simulink model "rlKinovaBallBalance"  (R2024a)
settings: Solver=ode15s  StartTime=0.0  StopTime=200  RelTol=1e-3  AbsTol=1e-3
undefined symbols (not defined in the file): ball, Control, L1, L2, L3, LS1, LS3, max_torque, plate, R1, R1_q0, R2, R2_q0, R3, R3_q0, R4_q0, R5_q0, Rover, rover_path, RS1, RS3, U0, X, Y, Z
libraries: sm_lib x227, nesl_utility x104, fl_lib x85, sdl_lib x20, nesl_utility_internal x17, ee_lib x10, mars_rover_lib x7, simulink x3, slpidlib x2, batteryecm_lib x2, robotalgslib x1, rllib x1
(part 3 of 10)

== system rlKinovaBallBalance/Kinova Ball Balance/7 DOF Manipulator/base_link ==
  Actuator1_AxisTransform : sm_lib/Frames and Transforms/Rigid Transform  RotationMethod=ArbitraryAxis  FollAlignAxisA=+X  BaseAlignAxisA=+Y  FollAlignAxisB=+Y  BaseAlignAxisB=+Z  RotationStandardAxis=+Z  RotationAngle=0  RotationAngleUnits=rad  RotationArbitraryAxis=[1, 0, 0]  RotationSequenceAxes=FollowerAxes  RotationSequence=XYX  RotationSequenceAngles=[0 0 0]  RotationSequenceAnglesUnits=deg  RotationMatrix=[1 0 0; 0 1 0; 0 0 1]  Quaternion=[1 0 0 0]  TranslationMethod=Cartesian  TranslationCartesianOffset=[0, 0, 0]  TranslationCartesianOffsetUnits=m  TranslationStandardAxis=+Z  TranslationStandardOffset=0  TranslationStandardOffsetUnits=m  TranslationROffset=0  TranslationROffsetUnits=m  TranslationThetaOffset=0  TranslationThetaOffsetUnits=deg  TranslationZOffset=0  TranslationZOffsetUnits=m
  Actuator1_OriginTransform : sm_lib/Frames and Transforms/Rigid Transform  RotationMethod=RotationSequence  FollAlignAxisA=+X  BaseAlignAxisA=+Y  FollAlignAxisB=+Y  BaseAlignAxisB=+Z  RotationStandardAxis=+Z  RotationAngle=0.0  RotationAngleUnits=deg  RotationArbitraryAxis=[0 0 1]  RotationSequenceAxes=BaseAxes  RotationSequence=XYZ  RotationSequenceAngles=[-3.141585307179587, 0, 0]  RotationSequenceAnglesUnits=rad  RotationMatrix=[1 0 0; 0 1 0; 0 0 1]  Quaternion=[1 0 0 0]  TranslationMethod=Cartesian  TranslationCartesianOffset=[0, 0, 0.15643]  TranslationCartesianOffsetUnits=m  TranslationStandardAxis=+Z  TranslationStandardOffset=0  TranslationStandardOffsetUnits=m  TranslationROffset=0  TranslationROffsetUnits=m  TranslationThetaOffset=0  TranslationThetaOffsetUnits=deg  TranslationZOffset=0  TranslationZOffsetUnits=m
  Base Link : Subsystem  Variant=on  VariantControlMode=label  VariantControl=Choice  LabelModeActiveChoice=Choice_1
  ReferenceFrame : sm_lib/Frames and Transforms/Reference Frame
  F : PMIOPort  Side=Left
  F1 : PMIOPort  Port=2  Side=Right
  connections:
  Actuator1_AxisTransform/RConn1 -- F1/RConn1
  Actuator1_AxisTransform/LConn1 -- Actuator1_OriginTransform/RConn1
  F/RConn1 -- Actuator1_OriginTransform/LConn1 -- ReferenceFrame/RConn1 -- Base Link/RConn1

== system rlKinovaBallBalance/Kinova Ball Balance/7 DOF Manipulator/mount ==
  Cylindrical Solid : sm_lib/Body Elements/Cylindrical Solid  CylinderRadius=0.1  CylinderRadiusUnits=m  CylinderLength=0.01  CylinderLengthUnits=m  ExportEntireGeometry=off  InertiaType=CalculateFromGeometry  BasedOnType=Density  Density=1000  DensityUnits=kg/m^3  Mass=1  MassUnits=kg  CenterOfMass=[0 0 0]  CenterOfMassUnits=m  MomentsOfInertia=[1 1 1]  MomentsOfInertiaUnits=kg*m^2  ProductsOfInertia=[0 0 0]  ProductsOfInertiaUnits=kg*m^2  GraphicType=FromGeometry  MarkerShape=Sphere  MarkerSize=10  GraphicVisPropType=SimpleVisualProperties  GraphicDiffuseColor=[0.6 0.6 0.6]  GraphicOpacity=1.0  GraphicSpecularColor=[0.5 0.5 0.5 1.0]  GraphicAmbientColor=[0.15 0.15 0.15 1.0]  GraphicEmissiveColor=[0.0 0.0 0.0 1.0]  GraphicShininess=75  DoExposeReferenceFrame=off  SerializedFrames=<Frames><Frame><Id>Frame1</Id><Value><Name>F1</Name><Origin><Source>GeometricFeature</Source><FeatureName>top surface</FeatureName></Origin><PrimaryAxis><DefinedDirection>+Z</DefinedDirection><Source>ReferenceFrame</Source><SourceDirection>+Z</SourceDirection><FeatureName></FeatureName></PrimaryAxis><SecondaryAxis><DefinedDirection>+X</DefinedDirection><Source>ReferenceFrame</Source><SourceDirection>+X</SourceDirection><FeatureName></FeatureName></SecondaryAxis></Value></Frame><Frame><Id>Frame2</Id><Value><Name>F2</Name><Origin><Source>GeometricFeature</Source><FeatureName>bottom surface</FeatureName></Origin><PrimaryAxis><DefinedDirection>+Z</DefinedDirection><Source>ReferenceFrame</Source><SourceDirection>+Z</SourceDirection><FeatureName></FeatureName></PrimaryAxis><SecondaryAxis><DefinedDirection>+X</DefinedDirection><Source>ReferenceFrame</Source><SourceDirection>+X</SourceDirection><FeatureName></FeatureName></SecondaryAxis></Value></Frame></Frames>
  F : PMIOPort  Side=Right
  F1 : PMIOPort  Port=2  Side=Left
  connections:
  Cylindrical Solid/LConn1 -- F1/RConn1
  F/RConn1 -- Cylindrical Solid/RConn1

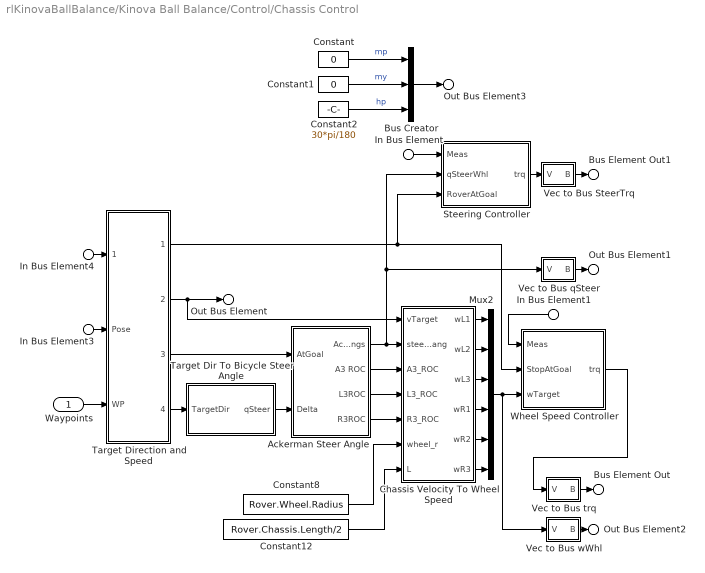
== system rlKinovaBallBalance/Kinova Ball Balance/Control/Chassis Control ==
  Waypoints : Inport
  In Bus Element1 : Inport  Port=2  PortName=Chassis  Element=Wheels.Drive
  In Bus Element : Inport  Port=2  PortName=Chassis  Element=Wheels.Steer
  In Bus Element3 : Inport  Port=3  PortName=Body  Element=Pose
  In Bus Element4 : Inport  Port=3  PortName=Body  Element=v
  Ackerman Steer Angle : Subsystem
  Bus Creator : BusCreator  Inputs=3
  Chassis Velocity To Wheel Speed : MATLAB Function  TreatAsAtomicUnit=on
  Constant : Constant  Value=0
  Constant1 : Constant  Value=0
  Constant12 : Constant  Value=Rover.Chassis.Length/2
  Constant2 : Constant  Value=30*pi/180
  Constant8 : Constant  Value=Rover.Wheel.Radius
  Mux2 : Mux  Inputs=6
  Steering Controller : Subsystem  mask{Kp=Control.Steer.Kp, Ki=Control.Steer.Ki, Kd=Control.Steer.Kd, N=Control.Steer.N, Ts_Targetq=Control.Steer.FiltTargetq, Ts_Measq=Control.Steer.FiltSensorq, trq_max_pos=Control.Steer.TrqCmdLimitPos, trq_max_neg=Control.Steer.TrqCmdLimitNeg}
      mask prompts: Kp "Propotional Gain"; Ki "Integral Gain"; Kd "Derivative Gain"; N "Filter Constant (derivative)"; Ts_Targetq "Target Angle (deg)"; Ts_Measq "Sensed Angle (deg)"; trq_max_pos "Torque Command Upper Limit (N*m)"; trq_max_neg "Torque Command Lower Limit (N*m)"
      mask DialogControl cont_pid Prompt: PID Controller
      mask DialogControl cont_filt_ts Prompt: Filter Time Constants
      mask DialogControl cont_trqCmdLim Prompt: Limits at Wheel
  Target Dir To Bicycle Steer Angle : Subsystem  mask{L=1, ld=0.75}
      mask prompts: L "Bicycle length"; ld "Lookahead distance"
      mask TypeOptions L: Bicycle length/Value
      mask TypeOptions ld: Lookahead distance/Value
  Target Direction and Speed : Subsystem
  Vec to Bus SteerTrq : Subsystem
  Vec to Bus qSteer : Subsystem
  Vec to Bus trq : Subsystem
  Vec to Bus wWhl : Subsystem
  Wheel Speed Controller : Subsystem  mask{Kp=Control.Drive.Kp, Ki=Control.Drive.Ki, Kd=Control.Drive.Kd, N=Control.Drive.N, Ts_Targetw=Control.Drive.FiltTargetw, Ts_Measw=Control.Drive.FiltSensorw, trq_max_pos=Control.Drive.TrqCmdLimitPos, trq_max_neg=Control.Drive.TrqCmdLimitNeg}
      mask prompts: Kp "Propotional Gain"; Ki "Integral Gain"; Kd "Derivative Gain"; N "Filter Constant (derivative)"; Ts_Targetw "Target Speed (sec)"; Ts_Measw "Sensed Speed (sec)"; trq_max_pos "Torque Command Upper Limit (N*m)"; trq_max_neg "Torque Command Lower Limit (N*m)"
      mask DialogControl Container4 Prompt: PID Controller
      mask DialogControl cont_filt_ts Prompt: Filter Time Constants
      mask DialogControl cont_trqCmdLim Prompt: Limits
  Bus Element Out1 : Outport  PortName=Ctrl  Element=Steer.trq
  Bus Element Out : Outport  PortName=Ctrl  Element=Drive.trq
  Out Bus Element : Outport  PortName=Ctrl  Element=Cmd.v
  Out Bus Element1 : Outport  PortName=Ctrl  Element=Cmd.qSteer
  Out Bus Element2 : Outport  PortName=Ctrl  Element=Cmd.wWhl
  Out Bus Element3 : Outport  PortName=Ctrl  Element=Camera
  wires:
  Chassis Velocity To Wheel Speed/6(wR3) -> Mux2/6
  Mux2/1 -> Wheel Speed Controller/3(wTarget), Vec to Bus wWhl/1(V)
  Ackerman Steer Angle/4(R3ROC) -> Chassis Velocity To Wheel Speed/5(R3_ROC)
  Chassis Velocity To Wheel Speed/5(wR2) -> Mux2/5
  Chassis Velocity To Wheel Speed/4(wR1) -> Mux2/4
  Ackerman Steer Angle/1(AckSteerAngs) -> Steering Controller/2(qSteerWhl), Vec to Bus qSteer/1(V), Chassis Velocity To Wheel Speed/2(steer_ang)
  Chassis Velocity To Wheel Speed/3(wL3) -> Mux2/3
  Constant12/1 -> Chassis Velocity To Wheel Speed/7(L)
  Constant8/1 -> Chassis Velocity To Wheel Speed/6(wheel_r)
  Chassis Velocity To Wheel Speed/2(wL2) -> Mux2/2
  Chassis Velocity To Wheel Speed/1(wL1) -> Mux2/1
  Ackerman Steer Angle/3(L3ROC) -> Chassis Velocity To Wheel Speed/4(L3_ROC)
  Ackerman Steer Angle/2(A3 ROC) -> Chassis Velocity To Wheel Speed/3(A3_ROC)
  Target Dir To Bicycle Steer Angle/1(qSteer) -> Ackerman Steer Angle/2(Delta)
  Wheel Speed Controller/1(trq) -> Vec to Bus trq/1(V)
  Steering Controller/1(trq) -> Vec to Bus SteerTrq/1(V)
  Vec to Bus trq/1(B) -> Bus Element Out/1
  Vec to Bus SteerTrq/1(B) -> Bus Element Out1/1
  In Bus Element1/1 -> Wheel Speed Controller/1(Meas)
  In Bus Element/1 -> Steering Controller/1(Meas)
  Vec to Bus qSteer/1(B) -> Out Bus Element1/1
  Vec to Bus wWhl/1(B) -> Out Bus Element2/1
  Target Direction and Speed/1(StopAtGoal) -> Wheel Speed Controller/2(StopAtGoal), Steering Controller/3(RoverAtGoal)
  Target Direction and Speed/2(vTarget) -> Chassis Velocity To Wheel Speed/1(vTarget), Out Bus Element/1
  In Bus Element3/1 -> Target Direction and Speed/2(Pose)
  Waypoints/1 -> Target Direction and Speed/3(WP)
  Target Direction and Speed/3(AtGoal) -> Ackerman Steer Angle/1(AtGoal)
  Target Direction and Speed/4(TargetDir) -> Target Dir To Bicycle Steer Angle/1(TargetDir)
  In Bus Element4/1 -> Target Direction and Speed/1(vRover)
  Constant/1 -> Bus Creator/1  "mp"
  Constant1/1 -> Bus Creator/2  "my"
  Constant2/1 -> Bus Creator/3  "hp"
  Bus Creator/1 -> Out Bus Element3/1

== system rlKinovaBallBalance/Kinova Ball Balance/Outputs/SelectSignal ==
  In Bus Element1 : Inport  PortName=C  Element=L1
  In Bus Element2 : Inport  PortName=C  Element=L2
  In Bus Element3 : Inport  PortName=C  Element=L3
  In Bus Element4 : Inport  PortName=C  Element=R1
  In Bus Element5 : Inport  PortName=C  Element=R2
  In Bus Element : Inport  PortName=C  Element=R3
  In Bus Element7 : Inport  Port=2  PortName=M  Element=w.L1
  In Bus Element10 : Inport  Port=2  PortName=M  Element=w.L2
  In Bus Element8 : Inport  Port=2  PortName=M  Element=w.L3
  In Bus Element11 : Inport  Port=2  PortName=M  Element=w.R3
  In Bus Element12 : Inport  Port=2  PortName=M  Element=w.R2
  In Bus Element9 : Inport  Port=2  PortName=M  Element=w.R1
  Mux{,1..5} (6 alike) : Mux  Inputs=2
  L1 : Outport
  L2 : Outport  Port=2
  L3 : Outport  Port=3
  R1 : Outport  Port=4
  R2 : Outport  Port=5
  R3 : Outport  Port=6
  wires:
  In Bus Element7/1 -> Mux/2  "Meas"
  Mux/1 -> L1/1
  In Bus Element1/1 -> Mux/1  "Cmd"
  In Bus Element2/1 -> Mux1/1  "Cmd"
  Mux1/1 -> L2/1
  In Bus Element10/1 -> Mux1/2  "Meas"
  In Bus Element8/1 -> Mux2/2  "Meas"
  Mux2/1 -> L3/1
  In Bus Element3/1 -> Mux2/1  "Cmd"
  In Bus Element4/1 -> Mux3/1  "Cmd"
  Mux3/1 -> R1/1
  In Bus Element9/1 -> Mux3/2  "Meas"
  In Bus Element12/1 -> Mux4/2  "Meas"
  Mux4/1 -> R2/1
  In Bus Element5/1 -> Mux4/1  "Cmd"
  In Bus Element/1 -> Mux5/1  "Cmd"
  Mux5/1 -> R3/1
  In Bus Element11/1 -> Mux5/2  "Meas"

== system rlKinovaBallBalance/Kinova Ball Balance/Outputs/SelectSignal1 ==
  In Bus Element1 : Inport  PortName=C  Element=L1
  In Bus Element3 : Inport  PortName=C  Element=L3
  In Bus Element4 : Inport  PortName=C  Element=R3
  In Bus Element2 : Inport  PortName=C  Element=R1
  In Bus Element5 : Inport  Port=2  PortName=M  Element=q.L1
  In Bus Element6 : Inport  Port=2  PortName=M  Element=q.L3
  In Bus Element7 : Inport  Port=2  PortName=M  Element=q.R1
  In Bus Element8 : Inport  Port=2  PortName=M  Element=q.R3
  Mux{,1..3} (4 alike) : Mux  Inputs=2
  L1 : Outport
  L3 : Outport  Port=2
  R1 : Outport  Port=3
  R3 : Outport  Port=4
  wires:
  In Bus Element8/1 -> Mux3/2  "Meas"
  Mux3/1 -> R3/1
  In Bus Element2/1 -> Mux2/1  "Cmd"
  In Bus Element4/1 -> Mux3/1  "Cmd"
  Mux2/1 -> R1/1
  In Bus Element7/1 -> Mux2/2  "Meas"
  In Bus Element6/1 -> Mux1/2  "Meas"
  Mux1/1 -> L3/1
  In Bus Element1/1 -> Mux/1  "Cmd"
  In Bus Element3/1 -> Mux1/1  "Cmd"
  Mux/1 -> L1/1
  In Bus Element5/1 -> Mux/2  "Meas"

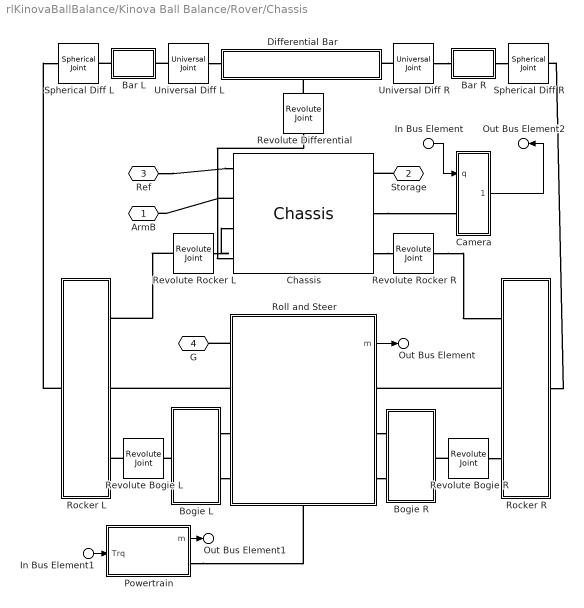
== system rlKinovaBallBalance/Kinova Ball Balance/Rover/Chassis ==
  In Bus Element1 : Inport  PortName=Ctrl
  In Bus Element : Inport  PortName=Ctrl  Element=Camera
  Bar L : Subsystem
  Bar R : Subsystem
  Bogie L : Subsystem
      mask Display: image('mars_rover_terrain_chassis_bogiel.png');
  Bogie R : Subsystem
      mask Display: image('mars_rover_terrain_chassis_bogier.png');
  Camera : Subsystem
      mask Display: image('mars_rover_terrain_chassis_camera.png')
  Chassis : mars_rover_lib/Chassis  body_opc=1
      link override RTG Bridge: Density=2000
      link override Rover Chassis: Density=1800
  Differential Bar : Subsystem
      settings: PortSchema="{\"entries\":[{\"content\":{\"sides\":[{\"content\":{\"connectorIds\":[\"LConn1\"]},\"type\":\"ConnectorPlacement.EquallySpacedRectSide\",\"uuid\":\"221cdbde-9b85-4491-b488-ab21b8b80dc6\"},{\"content\":{\"connectorIds\":[\"RConn1\"],\"side\":\"RIGHT\"},\"type\":\"ConnectorPlacement.EquallySpacedRectSide\",\"uuid\":\"70e1e311-dd19-4389-b9b6-0ef8a1761d4a\"},{\"content\":{\"connectorIds\":[],\"side\":\"TOP\"},\"type\":\"ConnectorPlacement.EquallySpacedRectSide\",\"uuid\":\"5e164d53-108c-4bd4-88ac-8f7d3d652b3e\"},{\"content\":{\"connectorIds\":[\"RConn2\"],\"side\":\"BOTTOM\"},\"type\":\"ConnectorPlacement.EquallySpacedRectSide\",\"uuid\":\"f6e2e044-5d94-4f88-a007-0ec3cd9ea455\"}]},\"type\":\"ConnectorPlacement.EquallySpacedConnector\",\"uuid\":\"e7d2f355-3189-4eee-a2bf-989eae5d727a\"}],\"packageUris\":[\"http://schema.mathworks.com/mf0/Connector/R2020b\"],\"version\":\"1.0\"}"
      mask Display: image('mars_rover_terrain_chassis_diffarm.png');
  Powertrain : Subsystem  Variant=on  VariantControlMode=label  VariantControl=Choice  LabelModeActiveChoice=Ideal  mask{popup_powertrain=Ideal}
      mask prompts: popup_powertrain "Powertrain Model"
      mask init:
      | set_param(gcb,'LabelModeActiveChoice',get_param(gcb,'popup_powertrain'));
      settings: AttributesFormatString=%<LabelModeActiveChoice>
      mask TypeOptions popup_powertrain: Ideal | Electrical
  Revolute Bogie L : sm_lib/Joints/Revolute Joint  JointMode=Normal  CompositeWrenchDir=FollowerOnBase  CompositeWrenchFrame=BaseFrame  SenseConstraintForce=off  SenseConstraintTorque=off  SenseTotalForce=off  SenseTotalTorque=off  PositionTargetSpecify=off  PositionTargetPriority=High  PositionTargetValue=0  PositionTargetValueUnits=deg  VelocityTargetSpecify=off  VelocityTargetPriority=High  VelocityTargetValue=0  VelocityTargetValueUnits=deg/s  EquilibriumPosition=0  EquilibriumPositionUnits=deg  SpringStiffness=0  SpringStiffnessUnits=N*m/deg  DampingCoefficient=0  DampingCoefficientUnits=N*m/(deg/s)  LowerLimitSpecify=off  LowerLimitBound=-90  LowerLimitBoundUnits=deg  LowerLimitStiffness=1e4  LowerLimitStiffnessUnits=N*m/deg  LowerLimitDamping=10  LowerLimitDampingUnits=N*m/(deg/s)  LowerLimitTransitionRegionWidth=0.1  LowerLimitTransitionRegionWidthUnits=deg  UpperLimitSpecify=off  UpperLimitBound=90  UpperLimitBoundUnits=deg  UpperLimitStiffness=1e4  UpperLimitStiffnessUnits=N*m/deg  UpperLimitDamping=10  UpperLimitDampingUnits=N*m/(deg/s)  UpperLimitTransitionRegionWidth=0.1  UpperLimitTransitionRegionWidthUnits=deg  TorqueActuationMode=NoTorque  MotionActuationMode=ComputedMotion  SensePosition=off  SenseVelocity=off  SenseAcceleration=off  SenseTorqueForce=off  SenseLowerLimitTorqueForce=off  SenseUpperLimitTorqueForce=off
  Revolute Bogie R : sm_lib/Joints/Revolute Joint  JointMode=Normal  CompositeWrenchDir=FollowerOnBase  CompositeWrenchFrame=BaseFrame  SenseConstraintForce=off  SenseConstraintTorque=off  SenseTotalForce=off  SenseTotalTorque=off  PositionTargetSpecify=off  PositionTargetPriority=High  PositionTargetValue=0  PositionTargetValueUnits=deg  VelocityTargetSpecify=off  VelocityTargetPriority=High  VelocityTargetValue=0  VelocityTargetValueUnits=deg/s  EquilibriumPosition=0  EquilibriumPositionUnits=deg  SpringStiffness=0  SpringStiffnessUnits=N*m/deg  DampingCoefficient=0  DampingCoefficientUnits=N*m/(deg/s)  LowerLimitSpecify=off  LowerLimitBound=-90  LowerLimitBoundUnits=deg  LowerLimitStiffness=1e4  LowerLimitStiffnessUnits=N*m/deg  LowerLimitDamping=10  LowerLimitDampingUnits=N*m/(deg/s)  LowerLimitTransitionRegionWidth=0.1  LowerLimitTransitionRegionWidthUnits=deg  UpperLimitSpecify=off  UpperLimitBound=90  UpperLimitBoundUnits=deg  UpperLimitStiffness=1e4  UpperLimitStiffnessUnits=N*m/deg  UpperLimitDamping=10  UpperLimitDampingUnits=N*m/(deg/s)  UpperLimitTransitionRegionWidth=0.1  UpperLimitTransitionRegionWidthUnits=deg  TorqueActuationMode=NoTorque  MotionActuationMode=ComputedMotion  SensePosition=off  SenseVelocity=off  SenseAcceleration=off  SenseTorqueForce=off  SenseLowerLimitTorqueForce=off  SenseUpperLimitTorqueForce=off
  Revolute Differential : sm_lib/Joints/Revolute Joint  JointMode=Normal  CompositeWrenchDir=FollowerOnBase  CompositeWrenchFrame=BaseFrame  SenseConstraintForce=off  SenseConstraintTorque=off  SenseTotalForce=off  SenseTotalTorque=off  PositionTargetSpecify=off  PositionTargetPriority=High  PositionTargetValue=45  PositionTargetValueUnits=deg  VelocityTargetSpecify=off  VelocityTargetPriority=High  VelocityTargetValue=1000  VelocityTargetValueUnits=deg/s  EquilibriumPosition=0  EquilibriumPositionUnits=deg  SpringStiffness=0  SpringStiffnessUnits=N*m/deg  DampingCoefficient=1e-3  DampingCoefficientUnits=N*m/(rad/s)  LowerLimitSpecify=off  LowerLimitBound=-90  LowerLimitBoundUnits=deg  LowerLimitStiffness=1e4  LowerLimitStiffnessUnits=N*m/deg  LowerLimitDamping=10  LowerLimitDampingUnits=N*m/(deg/s)  LowerLimitTransitionRegionWidth=0.1  LowerLimitTransitionRegionWidthUnits=deg  UpperLimitSpecify=off  UpperLimitBound=90  UpperLimitBoundUnits=deg  UpperLimitStiffness=1e4  UpperLimitStiffnessUnits=N*m/deg  UpperLimitDamping=10  UpperLimitDampingUnits=N*m/(deg/s)  UpperLimitTransitionRegionWidth=0.1  UpperLimitTransitionRegionWidthUnits=deg  TorqueActuationMode=NoTorque  MotionActuationMode=ComputedMotion  SensePosition=off  SenseVelocity=off  SenseAcceleration=off  SenseTorqueForce=off  SenseLowerLimitTorqueForce=off  SenseUpperLimitTorqueForce=off
  Revolute Rocker L : sm_lib/Joints/Revolute Joint  JointMode=Normal  CompositeWrenchDir=FollowerOnBase  CompositeWrenchFrame=BaseFrame  SenseConstraintForce=off  SenseConstraintTorque=off  SenseTotalForce=off  SenseTotalTorque=off  PositionTargetSpecify=on  PositionTargetPriority=Low  PositionTargetValue=90  PositionTargetValueUnits=deg  VelocityTargetSpecify=off  VelocityTargetPriority=High  VelocityTargetValue=5  VelocityTargetValueUnits=deg/s  EquilibriumPosition=0  EquilibriumPositionUnits=deg  SpringStiffness=0  SpringStiffnessUnits=N*m/deg  DampingCoefficient=0  DampingCoefficientUnits=N*m/(rad/s)  LowerLimitSpecify=off  LowerLimitBound=-90  LowerLimitBoundUnits=deg  LowerLimitStiffness=1e4  LowerLimitStiffnessUnits=N*m/deg  LowerLimitDamping=10  LowerLimitDampingUnits=N*m/(deg/s)  LowerLimitTransitionRegionWidth=0.1  LowerLimitTransitionRegionWidthUnits=deg  UpperLimitSpecify=off  UpperLimitBound=90  UpperLimitBoundUnits=deg  UpperLimitStiffness=1e4  UpperLimitStiffnessUnits=N*m/deg  UpperLimitDamping=10  UpperLimitDampingUnits=N*m/(deg/s)  UpperLimitTransitionRegionWidth=0.1  UpperLimitTransitionRegionWidthUnits=deg  TorqueActuationMode=NoTorque  MotionActuationMode=ComputedMotion  SensePosition=off  SenseVelocity=off  SenseAcceleration=off  SenseTorqueForce=off  SenseLowerLimitTorqueForce=off  SenseUpperLimitTorqueForce=off
  Revolute Rocker R : sm_lib/Joints/Revolute Joint  JointMode=Normal  CompositeWrenchDir=FollowerOnBase  CompositeWrenchFrame=BaseFrame  SenseConstraintForce=off  SenseConstraintTorque=off  SenseTotalForce=off  SenseTotalTorque=off  PositionTargetSpecify=on  PositionTargetPriority=Low  PositionTargetValue=-90  PositionTargetValueUnits=deg  VelocityTargetSpecify=off  VelocityTargetPriority=High  VelocityTargetValue=5  VelocityTargetValueUnits=deg/s  EquilibriumPosition=0  EquilibriumPositionUnits=deg  SpringStiffness=0  SpringStiffnessUnits=N*m/deg  DampingCoefficient=0  DampingCoefficientUnits=N*m/(rad/s)  LowerLimitSpecify=off  LowerLimitBound=-90  LowerLimitBoundUnits=deg  LowerLimitStiffness=1e4  LowerLimitStiffnessUnits=N*m/deg  LowerLimitDamping=10  LowerLimitDampingUnits=N*m/(deg/s)  LowerLimitTransitionRegionWidth=0.1  LowerLimitTransitionRegionWidthUnits=deg  UpperLimitSpecify=off  UpperLimitBound=90  UpperLimitBoundUnits=deg  UpperLimitStiffness=1e4  UpperLimitStiffnessUnits=N*m/deg  UpperLimitDamping=10  UpperLimitDampingUnits=N*m/(deg/s)  UpperLimitTransitionRegionWidth=0.1  UpperLimitTransitionRegionWidthUnits=deg  TorqueActuationMode=NoTorque  MotionActuationMode=ComputedMotion  SensePosition=off  SenseVelocity=off  SenseAcceleration=off  SenseTorqueForce=off  SenseLowerLimitTorqueForce=off  SenseUpperLimitTorqueForce=off
  Rocker L : Subsystem
      mask Display: image('mars_rover_terrain_chassis_rockerl.png');
  Rocker R : Subsystem
      mask Display: image('mars_rover_terrain_chassis_rockerr.png');
  Roll and Steer : Subsystem
      settings: PortSchema="{\"entries\":[{\"content\":{\"sides\":[{\"content\":{\"connectorIds\":[\"LConn1\",\"LConn2\",\"LConn3\",\"LConn4\"]},\"type\":\"ConnectorPlacement.EquallySpacedRectSide\",\"uuid\":\"a6cfb551-8d36-4b7b-a27d-860438164ad5\"},{\"content\":{\"connectorIds\":[\"Out1\",\"RConn1\",\"RConn2\",\"RConn3\"],\"side\":\"RIGHT\"},\"type\":\"ConnectorPlacement.EquallySpacedRectSide\",\"uuid\":\"63cd4134-c970-4875-8139-e10b865c9d5a\"},{\"content\":{\"connectorIds\":[],\"side\":\"TOP\"},\"type\":\"ConnectorPlacement.EquallySpacedRectSide\",\"uuid\":\"731de0f8-cd01-497c-8464-7874165ef328\"},{\"content\":{\"connectorIds\":[\"RConn4\"],\"side\":\"BOTTOM\"},\"type\":\"ConnectorPlacement.EquallySpacedRectSide\",\"uuid\":\"7e28c2ad-ee21-4cfa-8326-dce39ed3da54\"}]},\"type\":\"ConnectorPlacement.EquallySpacedConnector\",\"uuid\":\"7cc269d8-0205-4cd4-bd76-499a6cc04585\"}],\"packageUris\":[\"http://schema.mathworks.com/mf0/Connector/R2020b\"],\"version\":\"1.0\"}"
      mask Display: image('mars_rover_terrain_rollandsteer.png');
  Spherical Diff L : sm_lib/Joints/Spherical Joint  JointMode=Normal  CompositeWrenchDir=FollowerOnBase  CompositeWrenchFrame=BaseFrame  SenseConstraintForce=off  SenseConstraintTorque=off  SenseTotalForce=off  SenseTotalTorque=off  PositionTargetSpecify=off  PositionTargetPriority=High  PositionTargetRotationMethod=None  PositionTargetFollAlignAxisA=+X  PositionTargetBaseAlignAxisA=+Y  PositionTargetFollAlignAxisB=+Y  PositionTargetBaseAlignAxisB=+Z  PositionTargetRotationStandardAxis=+Z  PositionTargetRotationAngle=0.0  PositionTargetRotationAngleUnits=deg  PositionTargetRotationArbitraryAxis=[0 0 1]  PositionTargetRotationSequenceAxes=FollowerAxes  PositionTargetRotationSequence=XYX  PositionTargetRotationSequenceAngles=[0 0 0]  PositionTargetRotationSequenceAnglesUnits=deg  PositionTargetRotationMatrix=[1 0 0; 0 1 0; 0 0 1]  PositionTargetQuaternion=[1 0 0 0]  VelocityTargetSpecify=off  VelocityTargetPriority=High  VelocityTargetValue=[0 0 0]  VelocityTargetValueUnits=deg/s  VelocityTargetInFollowerFrame=on  EqPosRotationMethod=None  EqPosFollAlignAxisA=+X  EqPosBaseAlignAxisA=+Y  EqPosFollAlignAxisB=+Y  EqPosBaseAlignAxisB=+Z  EqPosRotationStandardAxis=+Z  EqPosRotationAngle=0.0  EqPosRotationAngleUnits=deg  EqPosRotationArbitraryAxis=[0 0 1]  EqPosRotationSequenceAxes=FollowerAxes  EqPosRotationSequence=XYX  EqPosRotationSequenceAngles=[0 0 0]  EqPosRotationSequenceAnglesUnits=deg  EqPosRotationMatrix=[1 0 0; 0 1 0; 0 0 1]  EqPosQuaternion=[1 0 0 0]  SpringStiffness=0  SpringStiffnessUnits=N*m/deg  DampingCoefficient=1e-3  DampingCoefficientUnits=N*m/(deg/s)  LowerLimitSpecify=off  LowerLimitBound=15  LowerLimitBoundUnits=deg  LowerLimitStiffness=1e4  LowerLimitStiffnessUnits=N*m/deg  LowerLimitDamping=10  LowerLimitDampingUnits=N*m/(deg/s)  LowerLimitTransitionRegionWidth=0.1  LowerLimitTransitionRegionWidthUnits=deg  UpperLimitSpecify=off  UpperLimitBound=45  UpperLimitBoundUnits=deg  UpperLimitStiffness=1e4  UpperLimitStiffnessUnits=N*m/deg  UpperLimitDamping=10  UpperLimitDampingUnits=N*m/(deg/s)  UpperLimitTransitionRegionWidth=0.1  UpperLimitTransitionRegionWidthUnits=deg  TorqueActuationMode=NoTorque  ActuateTorqueX=off  ActuateTorqueY=off  ActuateTorqueZ=off  ActuateTorque=off  ActuationFrame=BaseFrame  SensePosition=off  SenseVelocityX=off  SenseVelocityY=off  SenseVelocityZ=off  SenseVelocity=off  SenseAccelerationX=off  SenseAccelerationY=off  SenseAccelerationZ=off  SenseAcceleration=off  SenseLowerLimitTorqueMag=off  SenseUpperLimitTorqueMag=off  SensingFrame=BaseFrame
  Spherical Diff R : sm_lib/Joints/Spherical Joint  JointMode=Normal  CompositeWrenchDir=FollowerOnBase  CompositeWrenchFrame=BaseFrame  SenseConstraintForce=off  SenseConstraintTorque=off  SenseTotalForce=off  SenseTotalTorque=off  PositionTargetSpecify=off  PositionTargetPriority=High  PositionTargetRotationMethod=None  PositionTargetFollAlignAxisA=+X  PositionTargetBaseAlignAxisA=+Y  PositionTargetFollAlignAxisB=+Y  PositionTargetBaseAlignAxisB=+Z  PositionTargetRotationStandardAxis=+Z  PositionTargetRotationAngle=0.0  PositionTargetRotationAngleUnits=deg  PositionTargetRotationArbitraryAxis=[0 0 1]  PositionTargetRotationSequenceAxes=FollowerAxes  PositionTargetRotationSequence=XYX  PositionTargetRotationSequenceAngles=[0 0 0]  PositionTargetRotationSequenceAnglesUnits=deg  PositionTargetRotationMatrix=[1 0 0; 0 1 0; 0 0 1]  PositionTargetQuaternion=[1 0 0 0]  VelocityTargetSpecify=off  VelocityTargetPriority=High  VelocityTargetValue=[0 0 0]  VelocityTargetValueUnits=deg/s  VelocityTargetInFollowerFrame=on  EqPosRotationMethod=None  EqPosFollAlignAxisA=+X  EqPosBaseAlignAxisA=+Y  EqPosFollAlignAxisB=+Y  EqPosBaseAlignAxisB=+Z  EqPosRotationStandardAxis=+Z  EqPosRotationAngle=0.0  EqPosRotationAngleUnits=deg  EqPosRotationArbitraryAxis=[0 0 1]  EqPosRotationSequenceAxes=FollowerAxes  EqPosRotationSequence=XYX  EqPosRotationSequenceAngles=[0 0 0]  EqPosRotationSequenceAnglesUnits=deg  EqPosRotationMatrix=[1 0 0; 0 1 0; 0 0 1]  EqPosQuaternion=[1 0 0 0]  SpringStiffness=0  SpringStiffnessUnits=N*m/deg  DampingCoefficient=1e-3  DampingCoefficientUnits=N*m/(deg/s)  LowerLimitSpecify=off  LowerLimitBound=15  LowerLimitBoundUnits=deg  LowerLimitStiffness=1e4  LowerLimitStiffnessUnits=N*m/deg  LowerLimitDamping=10  LowerLimitDampingUnits=N*m/(deg/s)  LowerLimitTransitionRegionWidth=0.1  LowerLimitTransitionRegionWidthUnits=deg  UpperLimitSpecify=off  UpperLimitBound=45  UpperLimitBoundUnits=deg  UpperLimitStiffness=1e4  UpperLimitStiffnessUnits=N*m/deg  UpperLimitDamping=10  UpperLimitDampingUnits=N*m/(deg/s)  UpperLimitTransitionRegionWidth=0.1  UpperLimitTransitionRegionWidthUnits=deg  TorqueActuationMode=NoTorque  ActuateTorqueX=off  ActuateTorqueY=off  ActuateTorqueZ=off  ActuateTorque=off  ActuationFrame=BaseFrame  SensePosition=off  SenseVelocityX=off  SenseVelocityY=off  SenseVelocityZ=off  SenseVelocity=off  SenseAccelerationX=off  SenseAccelerationY=off  SenseAccelerationZ=off  SenseAcceleration=off  SenseLowerLimitTorqueMag=off  SenseUpperLimitTorqueMag=off  SensingFrame=BaseFrame
  Universal Diff L : sm_lib/Joints/Universal Joint  JointMode=Normal  CompositeWrenchDir=FollowerOnBase  CompositeWrenchFrame=BaseFrame  SenseConstraintForce=off  SenseConstraintTorque=off  SenseTotalForce=off  SenseTotalTorque=off  RxPositionTargetSpecify=off  RxPositionTargetPriority=High  RxPositionTargetValue=0  RxPositionTargetValueUnits=deg  RxVelocityTargetSpecify=off  RxVelocityTargetPriority=High  RxVelocityTargetValue=0  RxVelocityTargetValueUnits=deg/s  RxEquilibriumPosition=0  RxEquilibriumPositionUnits=deg  RxSpringStiffness=0  RxSpringStiffnessUnits=N*m/deg  RxDampingCoefficient=0  RxDampingCoefficientUnits=N*m/(rad/s)  RxLowerLimitSpecify=off  RxLowerLimitBound=-90  RxLowerLimitBoundUnits=deg  RxLowerLimitStiffness=1e4  RxLowerLimitStiffnessUnits=N*m/deg  RxLowerLimitDamping=10  RxLowerLimitDampingUnits=N*m/(deg/s)  RxLowerLimitTransitionRegionWidth=0.1  RxLowerLimitTransitionRegionWidthUnits=deg  RxUpperLimitSpecify=off  RxUpperLimitBound=90  RxUpperLimitBoundUnits=deg  RxUpperLimitStiffness=1e4  RxUpperLimitStiffnessUnits=N*m/deg  RxUpperLimitDamping=10  RxUpperLimitDampingUnits=N*m/(deg/s)  RxUpperLimitTransitionRegionWidth=0.1  RxUpperLimitTransitionRegionWidthUnits=deg  RxTorqueActuationMode=NoTorque  RxMotionActuationMode=ComputedMotion  RxSensePosition=off  RxSenseVelocity=off  RxSenseAcceleration=off  RxSenseTorqueForce=off  RxSenseLowerLimitTorqueForce=off  RxSenseUpperLimitTorqueForce=off  RyPositionTargetSpecify=off  RyPositionTargetPriority=High  RyPositionTargetValue=0  RyPositionTargetValueUnits=deg  RyVelocityTargetSpecify=off  RyVelocityTargetPriority=High  RyVelocityTargetValue=0  RyVelocityTargetValueUnits=deg/s  RyEquilibriumPosition=0  RyEquilibriumPositionUnits=deg  RySpringStiffness=0  RySpringStiffnessUnits=N*m/deg  RyDampingCoefficient=0  RyDampingCoefficientUnits=N*m/(rad/s)  RyLowerLimitSpecify=off  RyLowerLimitBound=-90  RyLowerLimitBoundUnits=deg  RyLowerLimitStiffness=1e4  RyLowerLimitStiffnessUnits=N*m/deg  RyLowerLimitDamping=10  RyLowerLimitDampingUnits=N*m/(deg/s)  RyLowerLimitTransitionRegionWidth=0.1  RyLowerLimitTransitionRegionWidthUnits=deg  RyUpperLimitSpecify=off  RyUpperLimitBound=90  RyUpperLimitBoundUnits=deg  RyUpperLimitStiffness=1e4  RyUpperLimitStiffnessUnits=N*m/deg  RyUpperLimitDamping=10  RyUpperLimitDampingUnits=N*m/(deg/s)  RyUpperLimitTransitionRegionWidth=0.1  RyUpperLimitTransitionRegionWidthUnits=deg  RyTorqueActuationMode=NoTorque  RyMotionActuationMode=ComputedMotion  RySensePosition=off  RySenseVelocity=off  RySenseAcceleration=off  RySenseTorqueForce=off  RySenseLowerLimitTorqueForce=off  RySenseUpperLimitTorqueForce=off
  Universal Diff R : sm_lib/Joints/Universal Joint  JointMode=Normal  CompositeWrenchDir=FollowerOnBase  CompositeWrenchFrame=BaseFrame  SenseConstraintForce=off  SenseConstraintTorque=off  SenseTotalForce=off  SenseTotalTorque=off  RxPositionTargetSpecify=off  RxPositionTargetPriority=High  RxPositionTargetValue=0  RxPositionTargetValueUnits=deg  RxVelocityTargetSpecify=off  RxVelocityTargetPriority=High  RxVelocityTargetValue=0  RxVelocityTargetValueUnits=deg/s  RxEquilibriumPosition=0  RxEquilibriumPositionUnits=deg  RxSpringStiffness=0  RxSpringStiffnessUnits=N*m/deg  RxDampingCoefficient=0  RxDampingCoefficientUnits=N*m/(rad/s)  RxLowerLimitSpecify=off  RxLowerLimitBound=-90  RxLowerLimitBoundUnits=deg  RxLowerLimitStiffness=1e4  RxLowerLimitStiffnessUnits=N*m/deg  RxLowerLimitDamping=10  RxLowerLimitDampingUnits=N*m/(deg/s)  RxLowerLimitTransitionRegionWidth=0.1  RxLowerLimitTransitionRegionWidthUnits=deg  RxUpperLimitSpecify=off  RxUpperLimitBound=90  RxUpperLimitBoundUnits=deg  RxUpperLimitStiffness=1e4  RxUpperLimitStiffnessUnits=N*m/deg  RxUpperLimitDamping=10  RxUpperLimitDampingUnits=N*m/(deg/s)  RxUpperLimitTransitionRegionWidth=0.1  RxUpperLimitTransitionRegionWidthUnits=deg  RxTorqueActuationMode=NoTorque  RxMotionActuationMode=ComputedMotion  RxSensePosition=off  RxSenseVelocity=off  RxSenseAcceleration=off  RxSenseTorqueForce=off  RxSenseLowerLimitTorqueForce=off  RxSenseUpperLimitTorqueForce=off  RyPositionTargetSpecify=off  RyPositionTargetPriority=High  RyPositionTargetValue=0  RyPositionTargetValueUnits=deg  RyVelocityTargetSpecify=off  RyVelocityTargetPriority=High  RyVelocityTargetValue=0  RyVelocityTargetValueUnits=deg/s  RyEquilibriumPosition=0  RyEquilibriumPositionUnits=deg  RySpringStiffness=0  RySpringStiffnessUnits=N*m/deg  RyDampingCoefficient=0  RyDampingCoefficientUnits=N*m/(rad/s)  RyLowerLimitSpecify=off  RyLowerLimitBound=-90  RyLowerLimitBoundUnits=deg  RyLowerLimitStiffness=1e4  RyLowerLimitStiffnessUnits=N*m/deg  RyLowerLimitDamping=10  RyLowerLimitDampingUnits=N*m/(deg/s)  RyLowerLimitTransitionRegionWidth=0.1  RyLowerLimitTransitionRegionWidthUnits=deg  RyUpperLimitSpecify=off  RyUpperLimitBound=90  RyUpperLimitBoundUnits=deg  RyUpperLimitStiffness=1e4  RyUpperLimitStiffnessUnits=N*m/deg  RyUpperLimitDamping=10  RyUpperLimitDampingUnits=N*m/(deg/s)  RyUpperLimitTransitionRegionWidth=0.1  RyUpperLimitTransitionRegionWidthUnits=deg  RyTorqueActuationMode=NoTorque  RyMotionActuationMode=ComputedMotion  RySensePosition=off  RySenseVelocity=off  RySenseAcceleration=off  RySenseTorqueForce=off  RySenseLowerLimitTorqueForce=off  RySenseUpperLimitTorqueForce=off
  ArmB : PMIOPort  Side=Left
  Storage : PMIOPort  Port=2  Side=Left
  Ref : PMIOPort  Port=3  Side=Left
  G : PMIOPort  Port=4  Side=Left
  Out Bus Element : Outport  PortName=m  Element=Wheels
  Out Bus Element1 : Outport  PortName=m  Element=Powertrain
  Out Bus Element2 : Outport  PortName=m  Element=Camera
  wires:
  Roll and Steer/1(m) -> Out Bus Element/1
  In Bus Element1/1 -> Powertrain/1(Trq)
  Powertrain/1(m) -> Out Bus Element1/1
  In Bus Element/1 -> Camera/1(q)
  Camera/1(m) -> Out Bus Element2/1
  connections:
  Ref/RConn1 -- Chassis/LConn1
  Revolute Rocker L/RConn1 -- Rocker L/RConn1
  Chassis/RConn3 -- Revolute Rocker R/LConn1
  Revolute Rocker L/LConn1 -- Chassis/LConn3
  Revolute Differential/LConn1 -- Chassis/LConn4
  Revolute Rocker R/RConn1 -- Rocker R/LConn1
  Revolute Differential/RConn1 -- Differential Bar/RConn2
  Rocker L/LConn1 -- Spherical Diff L/LConn1
  Rocker R/RConn1 -- Spherical Diff R/LConn1
  Rocker R/LConn2 -- Roll and Steer/RConn1
  Revolute Bogie R/LConn1 -- Rocker R/LConn3
  Chassis/LConn2 -- ArmB/RConn1
  Chassis/RConn2 -- Camera/LConn1
  Storage/RConn1 -- Chassis/RConn1
  Bogie L/RConn2 -- Roll and Steer/LConn4
  Bogie L/LConn1 -- Revolute Bogie L/RConn1
  Revolute Bogie R/RConn1 -- Bogie R/RConn1
  Roll and Steer/RConn2 -- Bogie R/LConn1
  Roll and Steer/RConn3 -- Bogie R/LConn2
  Roll and Steer/LConn1 -- G/RConn1
  Revolute Bogie L/LConn1 -- Rocker L/RConn3
  Roll and Steer/LConn2 -- Rocker L/RConn2
  Bogie L/RConn1 -- Roll and Steer/LConn3
  Powertrain/RConn1 -- Roll and Steer/RConn4
  Universal Diff L/RConn1 -- Bar L/LConn1
  Universal Diff L/LConn1 -- Differential Bar/LConn1
  Bar L/RConn1 -- Spherical Diff L/RConn1
  Universal Diff R/RConn1 -- Bar R/LConn1
  Universal Diff R/LConn1 -- Differential Bar/RConn1
  Bar R/RConn1 -- Spherical Diff R/RConn1

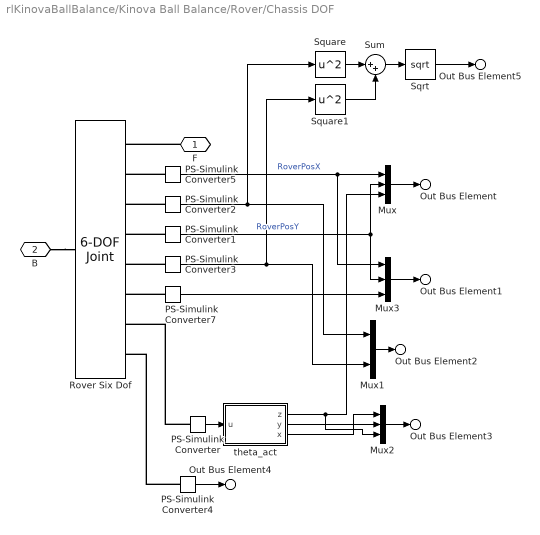
== system rlKinovaBallBalance/Kinova Ball Balance/Rover/Chassis DOF ==
  Mux : Mux  Inputs=3
  Mux1 : Mux  Inputs=2
  Mux2 : Mux  Inputs=3
  Mux3 : Mux  Inputs=3
  PS-Simulink Converter{,1..5,7} (7 alike) : nesl_utility/PS-Simulink Converter  PhysicalDomain=network_engine_domain  SubClassName=ps_output  LeftPortType=input  RightPortType=output  PseudoPeriodic=off  Frequencies=[]  VectorFormat=1-D array  Unit=inherit  AffineConversion=off
  Rover Six Dof : sm_lib/Joints/6-DOF Joint  JointMode=Normal  CompositeWrenchDir=FollowerOnBase  CompositeWrenchFrame=BaseFrame  SenseConstraintForce=off  SenseConstraintTorque=off  SenseTotalForce=off  SenseTotalTorque=off  PxPositionTargetSpecify=on  PxPositionTargetPriority=High  PxPositionTargetValue=x0  PxPositionTargetValueUnits=m  PxVelocityTargetSpecify=off  PxVelocityTargetPriority=High  PxVelocityTargetValue=0  PxVelocityTargetValueUnits=m/s  PxEquilibriumPosition=0  PxEquilibriumPositionUnits=m  PxSpringStiffness=0  PxSpringStiffnessUnits=N/m  PxDampingCoefficient=0  PxDampingCoefficientUnits=N/(m/s)  PxLowerLimitSpecify=off  PxLowerLimitBound=-1  PxLowerLimitBoundUnits=m  PxLowerLimitStiffness=1e6  PxLowerLimitStiffnessUnits=N/m  PxLowerLimitDamping=1e3  PxLowerLimitDampingUnits=N/(m/s)  PxLowerLimitTransitionRegionWidth=1e-4  PxLowerLimitTransitionRegionWidthUnits=m  PxUpperLimitSpecify=off  PxUpperLimitBound=1  PxUpperLimitBoundUnits=m  PxUpperLimitStiffness=1e6  PxUpperLimitStiffnessUnits=N/m  PxUpperLimitDamping=1e3  PxUpperLimitDampingUnits=N/(m/s)  PxUpperLimitTransitionRegionWidth=1e-4  PxUpperLimitTransitionRegionWidthUnits=m  PxTorqueActuationMode=NoTorque  PxMotionActuationMode=ComputedMotion  PxSensePosition=on  PxSenseVelocity=on  PxSenseAcceleration=off  PxSenseTorqueForce=off  PxSenseLowerLimitTorqueForce=off  PxSenseUpperLimitTorqueForce=off  PyPositionTargetSpecify=on  PyPositionTargetPriority=High  PyPositionTargetValue=y0  PyPositionTargetValueUnits=m  PyVelocityTargetSpecify=off  PyVelocityTargetPriority=High  PyVelocityTargetValue=-2  PyVelocityTargetValueUnits=m/s  PyEquilibriumPosition=0  PyEquilibriumPositionUnits=m  PySpringStiffness=0  PySpringStiffnessUnits=N/m  PyDampingCoefficient=0  PyDampingCoefficientUnits=N/(m/s)  PyLowerLimitSpecify=off  PyLowerLimitBound=-1  PyLowerLimitBoundUnits=m  PyLowerLimitStiffness=1e6  PyLowerLimitStiffnessUnits=N/m  PyLowerLimitDamping=1e3  PyLowerLimitDampingUnits=N/(m/s)  PyLowerLimitTransitionRegionWidth=1e-4  PyLowerLimitTransitionRegionWidthUnits=m  PyUpperLimitSpecify=off  PyUpperLimitBound=1  PyUpperLimitBoundUnits=m  PyUpperLimitStiffness=1e6  PyUpperLimitStiffnessUnits=N/m  PyUpperLimitDamping=1e3  PyUpperLimitDampingUnits=N/(m/s)  PyUpperLimitTransitionRegionWidth=1e-4  PyUpperLimitTransitionRegionWidthUnits=m  PyTorqueActuationMode=NoTorque  PyMotionActuationMode=ComputedMotion  PySensePosition=on  PySenseVelocity=on  PySenseAcceleration=off  PySenseTorqueForce=off  PySenseLowerLimitTorqueForce=off  PySenseUpperLimitTorqueForce=off  PzPositionTargetSpecify=on  PzPositionTargetPriority=High  PzPositionTargetValue=z0  PzPositionTargetValueUnits=m  PzVelocityTargetSpecify=off  PzVelocityTargetPriority=High  PzVelocityTargetValue=0  PzVelocityTargetValueUnits=m/s  PzEquilibriumPosition=0  PzEquilibriumPositionUnits=m  PzSpringStiffness=0  PzSpringStiffnessUnits=N/m  PzDampingCoefficient=0  PzDampingCoefficientUnits=N/(m/s)  PzLowerLimitSpecify=off  PzLowerLimitBound=-1  PzLowerLimitBoundUnits=m  PzLowerLimitStiffness=1e6  PzLowerLimitStiffnessUnits=N/m  PzLowerLimitDamping=1e3  PzLowerLimitDampingUnits=N/(m/s)  PzLowerLimitTransitionRegionWidth=1e-4  PzLowerLimitTransitionRegionWidthUnits=m  PzUpperLimitSpecify=off  PzUpperLimitBound=1  PzUpperLimitBoundUnits=m  PzUpperLimitStiffness=1e6  PzUpperLimitStiffnessUnits=N/m  PzUpperLimitDamping=1e3  PzUpperLimitDampingUnits=N/(m/s)  PzUpperLimitTransitionRegionWidth=1e-4  PzUpperLimitTransitionRegionWidthUnits=m  PzTorqueActuationMode=NoTorque  PzMotionActuationMode=ComputedMotion  PzSensePosition=on  PzSenseVelocity=off  PzSenseAcceleration=off  PzSenseTorqueForce=off  PzSenseLowerLimitTorqueForce=off  PzSenseUpperLimitTorqueForce=off  SphPositionTargetSpecify=on  SphPositionTargetPriority=High  SphPositionTargetRotationMethod=RotationSequence  SphPositionTargetFollAlignAxisA=+X  SphPositionTargetBaseAlignAxisA=+Y  SphPositionTargetFollAlignAxisB=+Y  SphPositionTargetBaseAlignAxisB=+Z  SphPositionTargetRotationStandardAxis=+X  SphPositionTargetRotationAngle=0.0647207  SphPositionTargetRotationAngleUnits=rad  SphPositionTargetRotationArbitraryAxis=[0.195566 -0.656945 0.728133]  SphPositionTargetRotationSequenceAxes=FollowerAxes  SphPositionTargetRotationSequence=ZYX  SphPositionTargetRotationSequenceAngles="[yaw0  pitch_0  roll_0]"  SphPositionTargetRotationSequenceAnglesUnits=rad  SphPositionTargetRotationMatrix=[1 0 0; 0 1 0; 0 0 1]  SphPositionTargetQuaternion=[1 0 0 0]  SphVelocityTargetSpecify=off  SphVelocityTargetPriority=High  SphVelocityTargetValue=[0 0 45]  SphVelocityTargetValueUnits=deg/s  SphVelocityTargetInFollowerFrame=on  SphEqPosRotationMethod=None  SphEqPosFollAlignAxisA=+X  SphEqPosBaseAlignAxisA=+Y  SphEqPosFollAlignAxisB=+Y  SphEqPosBaseAlignAxisB=+Z  SphEqPosRotationStandardAxis=+Z  SphEqPosRotationAngle=0.0  SphEqPosRotationAngleUnits=deg  SphEqPosRotationArbitraryAxis=[0 0 1]  SphEqPosRotationSequenceAxes=FollowerAxes  SphEqPosRotationSequence=XYX  SphEqPosRotationSequenceAngles=[0 0 0]  SphEqPosRotationSequenceAnglesUnits=deg  SphEqPosRotationMatrix=[1 0 0; 0 1 0; 0 0 1]  SphEqPosQuaternion=[1 0 0 0]  SphSpringStiffness=0  SphSpringStiffnessUnits=m*N/deg  SphDampingCoefficient=0  SphDampingCoefficientUnits=m*s*N/deg  SphLowerLimitSpecify=off  SphLowerLimitBound=15  SphLowerLimitBoundUnits=deg  SphLowerLimitStiffness=1e4  SphLowerLimitStiffnessUnits=N*m/deg  SphLowerLimitDamping=10  SphLowerLimitDampingUnits=N*m/(deg/s)  SphLowerLimitTransitionRegionWidth=0.1  SphLowerLimitTransitionRegionWidthUnits=deg  SphUpperLimitSpecify=off  SphUpperLimitBound=45  SphUpperLimitBoundUnits=deg  SphUpperLimitStiffness=1e4  SphUpperLimitStiffnessUnits=N*m/deg  SphUpperLimitDamping=10  SphUpperLimitDampingUnits=N*m/(deg/s)  SphUpperLimitTransitionRegionWidth=0.1  SphUpperLimitTransitionRegionWidthUnits=deg  SphTorqueActuationMode=NoTorque  SphActuateTorqueX=off  SphActuateTorqueY=off  SphActuateTorqueZ=off  SphActuateTorque=off  SphActuationFrame=BaseFrame  SphSensePosition=on  SphSenseVelocityX=off  SphSenseVelocityY=off  SphSenseVelocityZ=on  SphSenseVelocity=off  SphSenseAccelerationX=off  SphSenseAccelerationY=off  SphSenseAccelerationZ=off  SphSenseAcceleration=off  SphSenseLowerLimitTorqueMag=off  SphSenseUpperLimitTorqueMag=off  SphSensingFrame=BaseFrame
  Sqrt : Sqrt
  Square : Math  Operator=square
  Square1 : Math  Operator=square
  Sum : Sum  Inputs=|++
  theta_act : MATLAB Function  TreatAsAtomicUnit=on
  F : PMIOPort  Side=Right
  B : PMIOPort  Port=2  Side=Left
  Out Bus Element : Outport  PortName=m  Element=Pose
  Out Bus Element1 : Outport  PortName=m  Element=xyz
  Out Bus Element2 : Outport  PortName=m  Element=vxy
  Out Bus Element3 : Outport  PortName=m  Element=rpy
  Out Bus Element4 : Outport  PortName=m  Element=wz
  Out Bus Element5 : Outport  PortName=m  Element=v
  wires:
  theta_act/1(z) -> Mux2/3, Mux/3
  PS-Simulink Converter/1 -> theta_act/1(u)
  Mux2/1 -> Out Bus Element3/1
  Mux1/1 -> Out Bus Element2/1
  Mux3/1 -> Out Bus Element1/1
  PS-Simulink Converter7/1 -> Mux3/3
  theta_act/2(y) -> Mux2/2
  Mux/1 -> Out Bus Element/1
  PS-Simulink Converter5/1 -> Mux3/1, Mux/1  "RoverPosX"
  PS-Simulink Converter4/1 -> Out Bus Element4/1
  theta_act/3(x) -> Mux2/1
  PS-Simulink Converter1/1 -> Mux3/2, Mux/2  "RoverPosY"
  PS-Simulink Converter2/1 -> Square/1, Mux1/1
  Square1/1 -> Sum/2
  Square/1 -> Sum/1
  PS-Simulink Converter3/1 -> Square1/1, Mux1/2
  Sum/1 -> Sqrt/1
  Sqrt/1 -> Out Bus Element5/1
  connections:
  F/RConn1 -- Rover Six Dof/RConn1
  B/RConn1 -- Rover Six Dof/LConn1
  PS-Simulink Converter/LConn1 -- Rover Six Dof/RConn7
  PS-Simulink Converter4/LConn1 -- Rover Six Dof/RConn8
  PS-Simulink Converter5/LConn1 -- Rover Six Dof/RConn2
  PS-Simulink Converter1/LConn1 -- Rover Six Dof/RConn4
  PS-Simulink Converter7/LConn1 -- Rover Six Dof/RConn6
  PS-Simulink Converter2/LConn1 -- Rover Six Dof/RConn3
  PS-Simulink Converter3/LConn1 -- Rover Six Dof/RConn5

== system rlKinovaBallBalance/Kinova Ball Balance/Rover/Path ==
  Points : sm_lib/Curves and Surfaces/Point Cloud  CoordinatesMatrix=[rover_path.x rover_path.y rover_path.z]  CoordinatesMatrixUnits=m  GraphicType=MarkerCloud  GraphicSphereRadius=0.05*3  GraphicSphereRadiusUnits=m  GraphicVisPropType=SimpleVisualProperties  GraphicDiffuseColor=[0 0 1]  GraphicOpacity=1  GraphicSpecularColor=[0.5 0.5 0.5 1.0]  GraphicAmbientColor=[0.15 0.15 0.15 1.0]  GraphicEmissiveColor=[0.0 0.0 0.0 1.0]  GraphicShininess=75
  Rigid Transform : sm_lib/Frames and Transforms/Rigid Transform  RotationMethod=None  FollAlignAxisA=+X  BaseAlignAxisA=+Y  FollAlignAxisB=+Y  BaseAlignAxisB=+Z  RotationStandardAxis=+Z  RotationAngle=0.0  RotationAngleUnits=deg  RotationArbitraryAxis=[0 0 1]  RotationSequenceAxes=FollowerAxes  RotationSequence=XYX  RotationSequenceAngles=[0 0 0]  RotationSequenceAnglesUnits=deg  RotationMatrix=[1 0 0; 0 1 0; 0 0 1]  Quaternion=[1 0 0 0]  TranslationMethod=StandardAxis  TranslationCartesianOffset=[0 0 0]  TranslationCartesianOffsetUnits=m  TranslationStandardAxis=+Z  TranslationStandardOffset=rover_path.Offset_vis_z  TranslationStandardOffsetUnits=m  TranslationROffset=0  TranslationROffsetUnits=m  TranslationThetaOffset=0  TranslationThetaOffsetUnits=deg  TranslationZOffset=0  TranslationZOffsetUnits=m
  Spline : sm_lib/Curves and Surfaces/Spline  DataPoints=[rover_path.x rover_path.y rover_path.z]  DataPointsUnits=m  EndConditionType=Natural  GraphicType=FromGeometry  MarkerShape=Sphere  MarkerSize=10  GraphicVisPropType=SimpleVisualProperties  GraphicDiffuseColor=[0.1294 0.5333 0.8196]  GraphicOpacity=1  GraphicSpecularColor=[0.5 0.5 0.5 1.0]  GraphicAmbientColor=[0.15 0.15 0.15 1.0]  GraphicEmissiveColor=[0.0 0.0 0.0 1.0]  GraphicShininess=75
  R : PMIOPort  Side=Left
  connections:
  Points/LConn1 -- Rigid Transform/RConn1 -- Spline/LConn1
  R/RConn1 -- Rigid Transform/LConn1

== system rlKinovaBallBalance/Kinova Ball Balance/Rover/Terrain ==
  note: Uncomment for additional terrain visualization options.
  Contact : Subsystem  mask{contact_k=Rover.Wheel_Surface.Contact.k, contact_d=Rover.Wheel_Surface.Contact.d, contact_tw=Rover.Wheel_Surface.Contact.trans_depth, friction_mus=Rover.Wheel_Surface.Friction.mu_static, friction_mud=Rover.Wheel_Surface.Friction.mu_dynamic, friction_vcrit=Rover.Wheel_Surface.Friction.vel_crit}
      mask prompts: contact_k "Stiffness (N/m)"; contact_d "Damping (N/(m/s))"; contact_tw "Transition Region Width (m)"; friction_mus "Coefficient of Static Friction"; friction_mud "Coefficient of Dynamic Friction"; friction_vcrit "Critical Velocity (m/s)"
      mask DialogControl cont_contact Prompt: Contact Parameters
      mask DialogControl cont_friction Prompt: Contact Friction
  Terrain Geometry : sm_lib/Body Elements/File Solid  Commented=on  ExtGeomFileName=mars_terrain.stl  UnitType=Custom  ExtGeomFileUnits=m  StepReaderType=HEX  ExportConvexHullGeometry=off  InertiaType=CalculateFromGeometry  BasedOnType=Mass  Density=1000  DensityUnits=kg/m^3  Mass=1  MassUnits=kg  CenterOfMass=[0 0 0]  CenterOfMassUnits=m  MomentsOfInertia=[1 1 1]  MomentsOfInertiaUnits=kg*m^2  ProductsOfInertia=[0 0 0]  ProductsOfInertiaUnits=kg*m^2  GraphicType=FromGeometry  MarkerShape=Sphere  MarkerSize=10  GraphicVisPropType=SimpleVisualProperties  GraphicDiffuseColor=[1.0 0.6 0.6]  GraphicOpacity=1.0  GraphicSpecularColor=[0.5 0.5 0.5 1.0]  GraphicAmbientColor=[0.15 0.15 0.15 1.0]  GraphicEmissiveColor=[0.0 0.0 0.0 1.0]  GraphicShininess=75  DoExposeReferenceFrame=on  SerializedFrames=<Frames/>
  Terrain Point Cloud : sm_lib/Curves and Surfaces/Point Cloud  Commented=on  CoordinatesMatrix=mars_terrain_grid.ptcloud  CoordinatesMatrixUnits=m  GraphicType=MarkerCloud  GraphicSphereRadius=0.03  GraphicSphereRadiusUnits=m  GraphicVisPropType=SimpleVisualProperties  GraphicDiffuseColor=[0 1 0]  GraphicOpacity=1.0  GraphicSpecularColor=[0.5 0.5 0.5 1.0]  GraphicAmbientColor=[0.15 0.15 0.15 1.0]  GraphicEmissiveColor=[0.0 0.0 0.0 1.0]  GraphicShininess=75
  Terrain Grid Surface : sm_lib/Curves and Surfaces/Grid Surface  XGridVector=mars_terrain_grid.xg  XGridVectorUnits=m  YGridVector=mars_terrain_grid.yg  YGridVectorUnits=m  ZHeights=mars_terrain_grid.z_heights  ZHeightsUnits=m  GraphicType=FromGeometry  GraphicVisPropType=SimpleVisualProperties  GraphicDiffuseColor=[187 109 63]/255*1.3  GraphicOpacity=1  GraphicSpecularColor=[0.5 0.5 0.5 1.0]  GraphicAmbientColor=[0.15 0.15 0.15 1.0]  GraphicEmissiveColor=[0.0 0.0 0.0 1.0]  GraphicShininess=75
  W : PMIOPort  Side=Right
  G : PMIOPort  Port=2  Side=Right
  connections:
  W/RConn1 -- Terrain Point Cloud/LConn1 -- Terrain Geometry/RConn1 -- Terrain Grid Surface/LConn1
  Contact/RConn1 -- G/RConn1
  Contact/RConn2 -- Terrain Grid Surface/RConn1

== system rlKinovaBallBalance/Kinova Ball Balance/7 DOF Manipulator/Bracelet_Link/Bracelet Link ==
  FileSolid : Subsystem  VariantControl=Choice_1
  Inertia : Subsystem  VariantControl=Choice
  R : PMIOPort  Side=Right

== system rlKinovaBallBalance/Kinova Ball Balance/7 DOF Manipulator/ForeArm_Link/ForeArm Link ==
  FileSolid : Subsystem  VariantControl=Choice_1
  Inertia : Subsystem  VariantControl=Choice
  R : PMIOPort  Side=Right

== system rlKinovaBallBalance/Kinova Ball Balance/7 DOF Manipulator/HalfArm1_Link/HalfArm1 Link ==
  FileSolid : Subsystem  VariantControl=Choice_1
  Inertia : Subsystem  VariantControl=Choice
  R : PMIOPort  Side=Right

== system rlKinovaBallBalance/Kinova Ball Balance/7 DOF Manipulator/HalfArm2_Link/HalfArm2 Link ==
  FileSolid : Subsystem  VariantControl=Choice_1
  Inertia : Subsystem  VariantControl=Choice
  R : PMIOPort  Side=Right

== system rlKinovaBallBalance/Kinova Ball Balance/7 DOF Manipulator/Shoulder_Link/Shoulder Link ==
  FileSolid : Subsystem  VariantControl=Choice_1
  Inertia : Subsystem  VariantControl=Choice
  R : PMIOPort  Side=Right

== system rlKinovaBallBalance/Kinova Ball Balance/7 DOF Manipulator/Wrist1_Link/Wrist1 Link ==
  FileSolid : Subsystem  VariantControl=Choice_1
  Inertia : Subsystem  VariantControl=Choice
  R : PMIOPort  Side=Right

== system rlKinovaBallBalance/Kinova Ball Balance/7 DOF Manipulator/Wrist2_Link/Wrist2 Link ==
  FileSolid : Subsystem  VariantControl=Choice_1
  Inertia : Subsystem  VariantControl=Choice
  R : PMIOPort  Side=Right

== system rlKinovaBallBalance/Kinova Ball Balance/7 DOF Manipulator/base_link/Base Link ==
  FileSolid : Subsystem  VariantControl=Choice_1
  Inertia : Subsystem  VariantControl=Choice
  R : PMIOPort  Side=Right
